simulink model "main_observer_sim"  (R2015a)
settings: Solver=ode45  StartTime=0.0  StopTime=10  FixedStep=1e-4  MaxStep=1e-3  RelTol=1e-3
values from neighbouring files (symbols this model uses):
  A = [-1.27797343778 0.333872204357 1.75620734089 -1.56224484389 -1.03731554325 1.61047691587 -0.301778945187 -0.746429865998 -1.0138823557 1.30543582149 -0.0889326780489 0.0332636291631 ... (36 elements, 6x6)]    [A.mat]    (also in main_Observer.m = sys_rand.A)
  C = [0.8954663563 -0.344571536199 -1.3867839766 0 0 -1.25274492024 0.0740580691775 -0.828704014931 -0.552438671582 0 -0.23750602142 -0.378709097599 ... (18 elements, 3x6)]    [C.mat]    (also in main_Observer.m = sys_rand.C)
  Gama = eta*A-X*C    [main_Observer.m]    (also in observer.mat = [22.8246151403 -1331.98593789 -219.710031357 145.030296815 2)
  H = [0.574066719729 0.519875550069 -0.636819062075 -0.770886938571 0.309777205751 -0.804844094201]    [H.mat]    (also in main_Observer.m = B(:,end))
  Phi = inv(delta1)*Phi_hat    [main_Observer.m]    (also in observer.mat = [35.9769844985 416.30041215 22.0641801854 39.341911218 -79.7)
  theta = theta1+Y*theta2    [main_Observer.m]    (also in observer.mat = [0.23961688316 -297.740368665 3.95476908974 -0.24732331029 -)
settings Model: Creator=p4wp4w  LastModifiedBy=p4wp4w

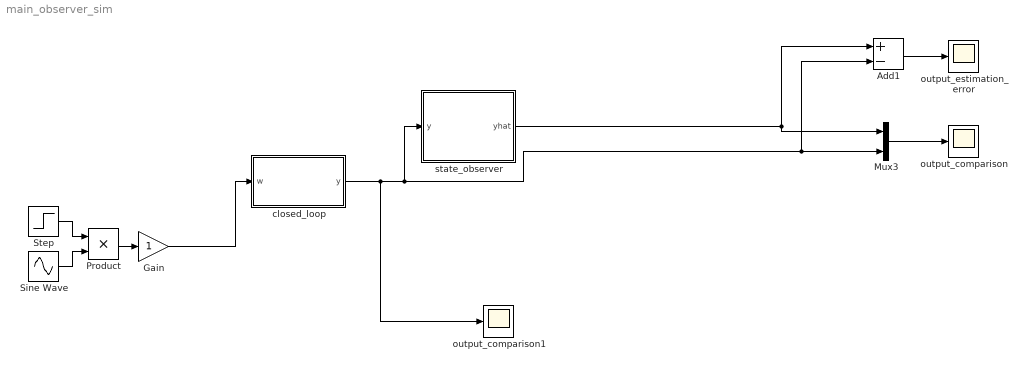
== system main_observer_sim ==
  Add1 : Sum  Inputs=+-
  Gain : Gain
  Mux3 : Mux  Inputs=2
  Product : Product
  Sine Wave : Sin  Frequency=10  SampleTime=0
  Step : Step  Before=8  After=0  SampleTime=0
  closed_loop : Subsystem
  output_comparison : Scope
      settings: YMin=-0.0024  YMax=-2.1684e-19
  output_comparison1 : Scope
      settings: YMin=-0.0024  YMax=-2.1684e-19  SaveName=ScopeData5
  output_estimation_error : Scope
      settings: YMin=-0.0024  YMax=-2.1684e-19  SaveName=ScopeData3
  state_observer : Subsystem
  wires:
  closed_loop/1(y) -> output_comparison1/1, Add1/2, Mux3/2, state_observer/1(y)
  Mux3/1 -> output_comparison/1
  state_observer/1(yhat) -> Mux3/1, Add1/1
  Gain/1 -> closed_loop/1(w)
  Add1/1 -> output_estimation_error/1
  Product/1 -> Gain/1
  Step/1 -> Product/1
  Sine Wave/1 -> Product/2

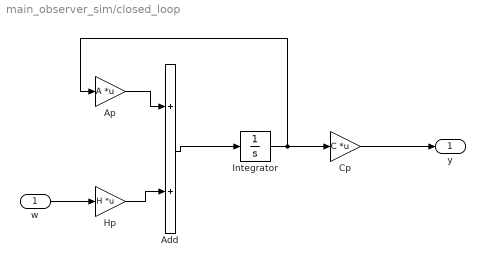
== system main_observer_sim/closed_loop ==
  w : Inport
  Add : Sum
  Ap : Gain  Gain=A  Multiplication=Matrix(K*u)
  Cp : Gain  Gain=C  Multiplication=Matrix(K*u)
  Hp : Gain  Gain=H  Multiplication=Matrix(K*u)
  Integrator : Integrator
  y : Outport
  wires:
  w/1 -> Hp/1
  Add/1 -> Integrator/1
  Integrator/1 -> Cp/1, Ap/1
  Ap/1 -> Add/1
  Hp/1 -> Add/2
  Cp/1 -> y/1

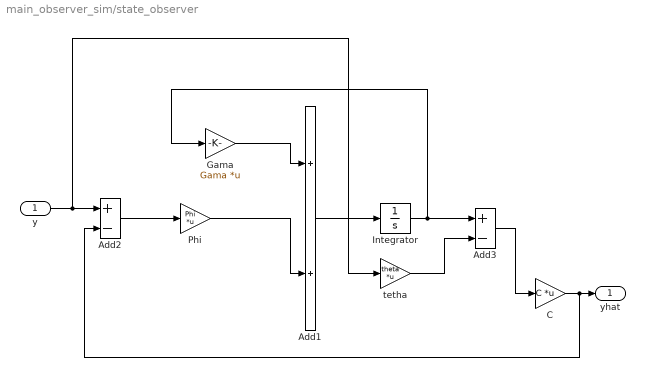
== system main_observer_sim/state_observer ==
  y : Inport
  Add1 : Sum
  Add2 : Sum  Inputs=+-
  Add3 : Sum  Inputs=+-
  C : Gain  Gain=C  Multiplication=Matrix(K*u)
  Gama : Gain  Gain=Gama  Multiplication=Matrix(K*u)
  Integrator : Integrator
  Phi : Gain  Gain=Phi  Multiplication=Matrix(K*u)
  tetha : Gain  Gain=theta  Multiplication=Matrix(K*u)
  yhat : Outport
  wires:
  y/1 -> tetha/1, Add2/1
  C/1 -> Add2/2, yhat/1
  Add1/1 -> Integrator/1
  Gama/1 -> Add1/1
  Integrator/1 -> Gama/1, Add3/1
  Phi/1 -> Add1/2
  Add2/1 -> Phi/1
  tetha/1 -> Add3/2
  Add3/1 -> C/1
